simulink model "compare"  (R2018b)
settings: Solver=ode45  StartTime=0.0  StopTime=100  RelTol=1e-3
libraries: neural x79
(part 4 of 4)

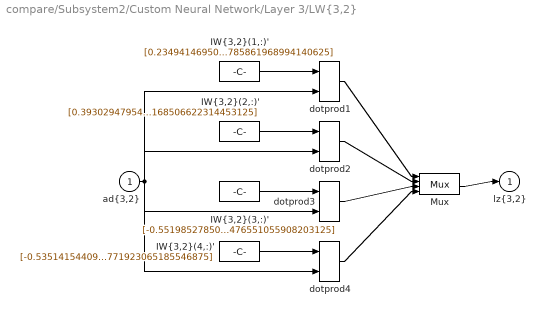
== system compare/Subsystem2/Custom Neural Network/Layer 3/LW{3,2} ==
  "ad{3,2}" : Inport  PortDimensions=15  SampleTime=1
      mask Display: e = 0.06;c1 = [120 230 180]/255;c2 = ([120 230 180]+0)/(256+128);c3 = ([120 230 180]+128)/(256+128);patch([0 1 1 0],[0 0 1 1],c1);patch([0 1 1 1-e 1-e 0+e],[0 0 1 1-e 0+e 0+e],c2);patch([0 0 1 1-e 0+e 0+e],[0 1 1 1-e 1-e 0+e],c3);plot([0 1 1 0 0],[0 0 1 1 0]);
  "IW{3,2}(1,:)'" : Constant  Value=[0.2349414695043779699457076048929593525826930999755859375;-0.308873157166934697581694990731193684041500091552734375;0.004868031555572019906941161337954326882027089595794677734375;-0.691927257149973495842232296126894652843475341796875;0.59437512293096628201993780749035067856311798095703125;0.262904797051506211591487272016820497810840606689453125;-0.5764385735392842935453927566413767635822296142578125;-0.36726365206025646248377825031639076769351959228515625;0.07868494933792673229344671881335671059787273406982421875;0.1470371649624575283166194594741682521998882293701171875;0.2430770873424570321930104910279624164104461669921875;0.41449358131859115328410325673758052289485931396484375;0.76203687536312092465351497594383545219898223876953125;-0.1882893600816501755712550902899238280951976776123046875;-0.039043678194928578550904063604320981539785861968994140625]
      mask Display: e = 0.06;c1 = [120 150 230]/255;c2 = ([120 150 230]+0)/383;c3 = ([120 150 230]+128)/383;patch([0 1 1 0],[0 0 1 1],c1);patch([0 1 1 1-e 1-e 0+e],[0 0 1 1-e 0+e 0+e],c2);patch([0 0 1 1-e 0+e 0+e],[0 1 1 1-e 1-e 0+e],c3);plot([0 1 1 0 0],[0 0 1 1 0]);disp('weights');
  "IW{3,2}(2,:)'" : Constant  Value=[0.39302947954107370076570759920286945998668670654296875;0.323308783750280215318895216114469803869724273681640625;0.050762973307179902471286681020501418970525264739990234375;0.0278888101955697374767506602211142308078706264495849609375;0.57850250684399029399429537079413421452045440673828125;-0.5850420064040349199530055557261221110820770263671875;0.240563216588854544841780125352670438587665557861328125;0.35353039090871785088410206299158744513988494873046875;0.375144878673505599575577207360765896737575531005859375;-0.06293451133035622702127653838033438660204410552978515625;0.50526278618238273931950743644847534596920013427734375;-0.627505336970902050097720348276197910308837890625;0.374106027913270688944891162464045919477939605712890625;0.352272400218531178683889493186143226921558380126953125;0.52316346319008222298663213223335333168506622314453125]
      mask Display: e = 0.06;c1 = [120 150 230]/255;c2 = ([120 150 230]+0)/383;c3 = ([120 150 230]+128)/383;patch([0 1 1 0],[0 0 1 1],c1);patch([0 1 1 1-e 1-e 0+e],[0 0 1 1-e 0+e 0+e],c2);patch([0 0 1 1-e 0+e 0+e],[0 1 1 1-e 1-e 0+e],c3);plot([0 1 1 0 0],[0 0 1 1 0]);disp('weights');
  "IW{3,2}(3,:)'" : Constant  Value=[-0.5519852785056382771244898322038352489471435546875;0.362949217835002835297331102992757223546504974365234375;-0.38966535730814533255994547289446927607059478759765625;-0.390442448661180330216069478410645388066768646240234375;-0.2078762341590312534567175362099078483879566192626953125;-0.1987820843011612048645275763192330487072467803955078125;-0.6103199035883493106524610993801616132259368896484375;-0.4000337082474556549271937910816632211208343505859375;-0.2016597369327599309496434898392180912196636199951171875;0.045040858824803096938094171264310716651380062103271484375;-0.5907081449059508049259648032602854073047637939453125;0.4155974330540705974357251761830411851406097412109375;0.257777521402553666529655629346962086856365203857421875;-0.6087282204211990066511361874290741980075836181640625;-0.0250695617602581972971353962975626927800476551055908203125]
      mask Display: e = 0.06;c1 = [120 150 230]/255;c2 = ([120 150 230]+0)/383;c3 = ([120 150 230]+128)/383;patch([0 1 1 0],[0 0 1 1],c1);patch([0 1 1 1-e 1-e 0+e],[0 0 1 1-e 0+e 0+e],c2);patch([0 0 1 1-e 0+e 0+e],[0 1 1 1-e 1-e 0+e],c3);plot([0 1 1 0 0],[0 0 1 1 0]);disp('weights');
  "IW{3,2}(4,:)'" : Constant  Value=[-0.53514154409166747594639446106157265603542327880859375;0.045934037007529703033892332086907117627561092376708984375;0.00922527512755755806084234649233621894381940364837646484375;-0.71782457172495750530316627191496081650257110595703125;-0.6016298104210184849449660760001279413700103759765625;-0.353988558186288881923786675542942248284816741943359375;-0.0155942267474686417638718438638534280471503734588623046875;0.387524036026416440758879389250068925321102142333984375;-0.8661200883669859518221301186713390052318572998046875;0.098478188126410959313261628267355263233184814453125;0.226152763400829182049989185543381609022617340087890625;-0.35104978190615288013987083104439079761505126953125;0.607123351414204481812930680462159216403961181640625;-0.28884339849374740527565563752432353794574737548828125;-0.58973522060840632974532127263955771923065185546875]
      mask Display: e = 0.06;c1 = [120 150 230]/255;c2 = ([120 150 230]+0)/383;c3 = ([120 150 230]+128)/383;patch([0 1 1 0],[0 0 1 1],c1);patch([0 1 1 1-e 1-e 0+e],[0 0 1 1-e 0+e 0+e],c2);patch([0 0 1 1-e 0+e 0+e],[0 1 1 1-e 1-e 0+e],c3);plot([0 1 1 0 0],[0 0 1 1 0]);disp('weights');
  Mux : Mux
      mask Display: e = 0.06;c1 = [120 150 230]/255;c2 = ([120 150 230]+0)/383;c3 = ([120 150 230]+128)/383;patch([0 1 1 0],[0 0 1 1],c1);patch([0 1 1 1-e 1-e 0+e],[0 0 1 1-e 0+e 0+e],c2);patch([0 0 1 1-e 0+e 0+e],[0 1 1 1-e 1-e 0+e],c3);plot([0 1 1 0 0],[0 0 1 1 0]);disp('Mux');
  dotprod{1..4} (4 alike) : neural/Weight Functions/dotprod
  "lz{3,2}" : Outport
      mask Display: e = 0.06;c1 = [120 230 180]/255;c2 = ([120 230 180]+0)/(256+128);c3 = ([120 230 180]+128)/(256+128);patch([0 1 1 0],[0 0 1 1],c1);patch([0 1 1 1-e 1-e 0+e],[0 0 1 1-e 0+e 0+e],c2);patch([0 0 1 1-e 0+e 0+e],[0 1 1 1-e 1-e 0+e],c3);plot([0 1 1 0 0],[0 0 1 1 0]);
  wires:
  "IW{3,2}(1,:)'"/1 -> dotprod1/1
  "ad{3,2}"/1 -> dotprod1/2, dotprod2/2, dotprod3/2, dotprod4/2
  dotprod1/1 -> Mux/1
  "IW{3,2}(2,:)'"/1 -> dotprod2/1
  dotprod2/1 -> Mux/2
  "IW{3,2}(3,:)'"/1 -> dotprod3/1
  dotprod3/1 -> Mux/3
  "IW{3,2}(4,:)'"/1 -> dotprod4/1
  dotprod4/1 -> Mux/4
  Mux/1 -> "lz{3,2}"/1
